simulink model "P2002_230207_MasterTest01"  (R2022b)
settings: Solver=VariableStepAuto  StartTime=0.0  StopTime=30  RelTol=1e-7
settings Model: PacingRate=0.100000  Creator=turib  LastModifiedBy=turib

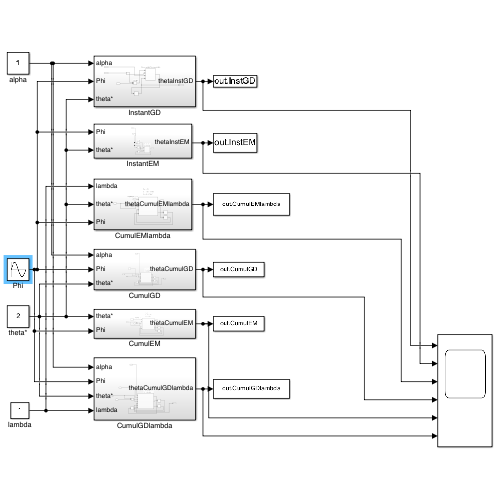
[thumbnail: Simulink's stored preview of the top-level diagram]
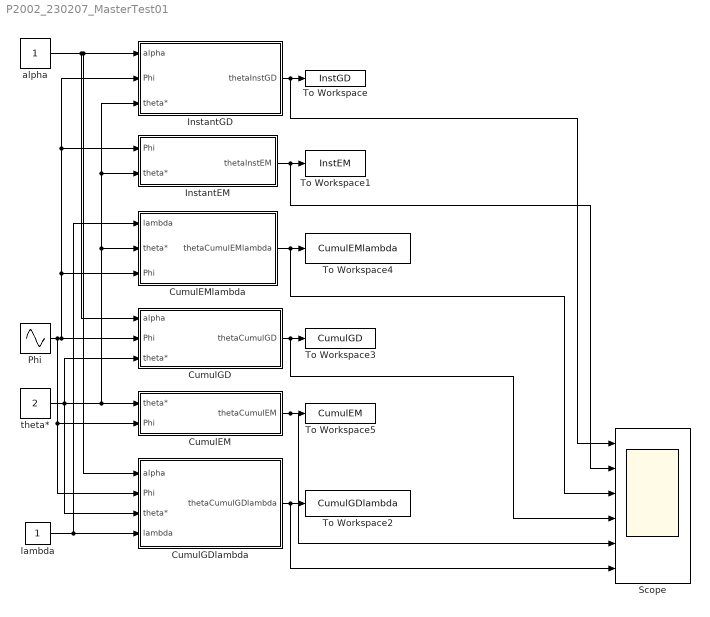
== system P2002_230207_MasterTest01 ==
  CumulEM : Subsystem
  CumulEMlambda : Subsystem
  CumulGD : Subsystem
  CumulGDlambda : Subsystem
  InstantEM : Subsystem
  InstantGD : Subsystem
  Phi : Sin  SampleTime=0
  Scope : Scope  NumInputPorts=6
  To Workspace : ToWorkspace  VariableName=InstGD  SampleTime=-1
  To Workspace1 : ToWorkspace  VariableName=InstEM  SampleTime=-1
  To Workspace2 : ToWorkspace  VariableName=CumulGDlambda  SampleTime=-1
  To Workspace3 : ToWorkspace  VariableName=CumulGD  SampleTime=-1
  To Workspace4 : ToWorkspace  VariableName=CumulEMlambda  SampleTime=-1
  To Workspace5 : ToWorkspace  VariableName=CumulEM  SampleTime=-1
  alpha : Constant
  lambda : Constant
  theta* : Constant  Value=2
  wires:
  lambda/1 -> CumulGDlambda/4(lambda), CumulEMlambda/1(lambda)
  alpha/1 -> InstantGD/1(alpha), CumulGDlambda/1(alpha), CumulGD/1(alpha)
  Phi/1 -> CumulEM/2(Phi), CumulGDlambda/2(Phi), CumulGD/2(Phi), InstantGD/2(Phi), InstantEM/1(Phi), CumulEMlambda/3(Phi)
  theta*/1 -> CumulGDlambda/3(theta*), InstantEM/2(theta*), InstantGD/3(theta*), CumulEMlambda/2(theta*), CumulEM/1(theta*), CumulGD/3(theta*)
  CumulEMlambda/1(thetaCumulEMlambda) -> Scope/3, To Workspace4/1
  InstantGD/1(thetaInstGD) -> Scope/1, To Workspace/1
  InstantEM/1(thetaInstEM) -> Scope/2, To Workspace1/1
  CumulGD/1(thetaCumulGD) -> Scope/4, To Workspace3/1
  CumulEM/1(thetaCumulEM) -> Scope/5, To Workspace5/1
  CumulGDlambda/1(thetaCumulGDlambda) -> Scope/6, To Workspace2/1

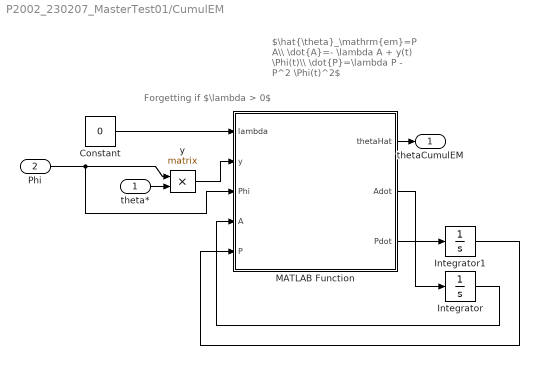
== system P2002_230207_MasterTest01/CumulEM ==
  note: $\hat{\theta}_\mathrm{em}=P A\\ \dot{A}=- \lambda A + y(t) \Phi(t)\\ \dot{P}=\lambda P - P^2 \Phi(t)^2$
  note: Forgetting if $\lambda > 0$
  theta* : Inport
  Phi : Inport  Port=2
  Constant : Constant  Value=0
  Integrator : Integrator  InitialCondition=1
  Integrator1 : Integrator  InitialCondition=1
  MATLAB Function : MATLAB Function  TreatAsAtomicUnit=on
  y : Product  Multiplication=Matrix(*)  OutDataTypeStr=double
  thetaCumulEM : Outport
  wires:
  theta*/1 -> y/2
  MATLAB Function/3(Pdot) -> Integrator1/1
  Integrator1/1 -> MATLAB Function/5(P)
  Integrator/1 -> MATLAB Function/4(A)
  Constant/1 -> MATLAB Function/1(lambda)
  y/1 -> MATLAB Function/2(y)
  MATLAB Function/2(Adot) -> Integrator/1
  MATLAB Function/1(thetaHat) -> thetaCumulEM/1
  Phi/1 -> y/1, MATLAB Function/3(Phi)

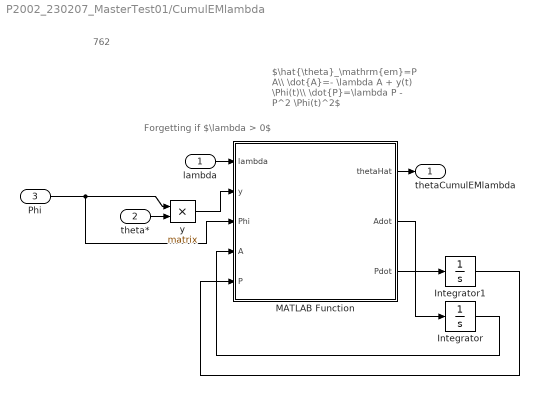
== system P2002_230207_MasterTest01/CumulEMlambda ==
  note: 762
  note: $\hat{\theta}_\mathrm{em}=P A\\ \dot{A}=- \lambda A + y(t) \Phi(t)\\ \dot{P}=\lambda P - P^2 \Phi(t)^2$
  note: Forgetting if $\lambda > 0$
  lambda : Inport
  theta* : Inport  Port=2
  Phi : Inport  Port=3
  Integrator : Integrator  InitialCondition=1
  Integrator1 : Integrator  InitialCondition=1
  MATLAB Function : MATLAB Function  TreatAsAtomicUnit=on
  y : Product  Multiplication=Matrix(*)  OutDataTypeStr=double
  thetaCumulEMlambda : Outport
  wires:
  theta*/1 -> y/2
  MATLAB Function/3(Pdot) -> Integrator1/1
  Integrator1/1 -> MATLAB Function/5(P)
  Integrator/1 -> MATLAB Function/4(A)
  lambda/1 -> MATLAB Function/1(lambda)
  y/1 -> MATLAB Function/2(y)
  MATLAB Function/2(Adot) -> Integrator/1
  MATLAB Function/1(thetaHat) -> thetaCumulEMlambda/1
  Phi/1 -> y/1, MATLAB Function/3(Phi)

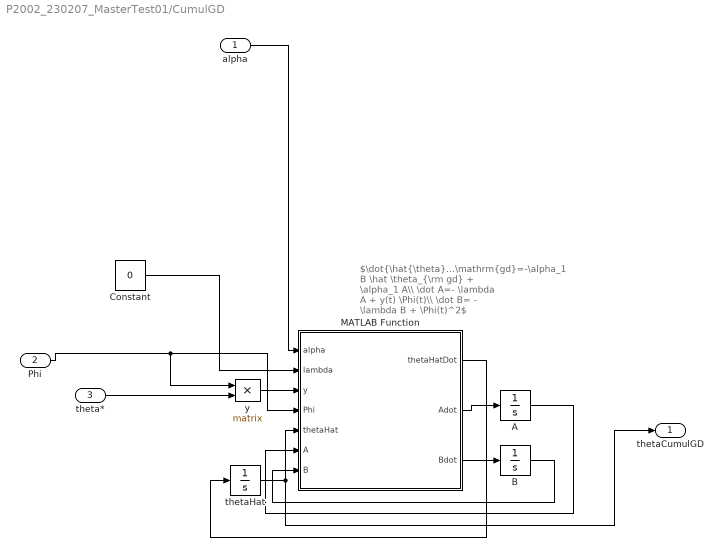
== system P2002_230207_MasterTest01/CumulGD ==
  note: $\dot{\hat{\theta}}_\mathrm{gd}=-\alpha_1 B \hat \theta_{\rm gd} + \alpha_1 A\\ \dot A=- \lambda A + y(t) \Phi(t)\\ \dot B= - \lambda B + \Phi(t)^2$
  alpha : Inport
  Phi : Inport  Port=2
  theta* : Inport  Port=3
  A : Integrator  InitialCondition=1
  B : Integrator  InitialCondition=1
  Constant : Constant  Value=0
  MATLAB Function : MATLAB Function  TreatAsAtomicUnit=on
  thetaHat : Integrator
  y : Product  Multiplication=Matrix(*)  OutDataTypeStr=double
  thetaCumulGD : Outport
  wires:
  thetaHat/1 -> thetaCumulGD/1, MATLAB Function/5(thetaHat)
  B/1 -> MATLAB Function/7(B)
  MATLAB Function/3(Bdot) -> B/1
  A/1 -> MATLAB Function/6(A)
  theta*/1 -> y/2
  MATLAB Function/1(thetaHatDot) -> thetaHat/1
  y/1 -> MATLAB Function/3(y)
  MATLAB Function/2(Adot) -> A/1
  Phi/1 -> MATLAB Function/4(Phi), y/1
  alpha/1 -> MATLAB Function/1(alpha)
  Constant/1 -> MATLAB Function/2(lambda)

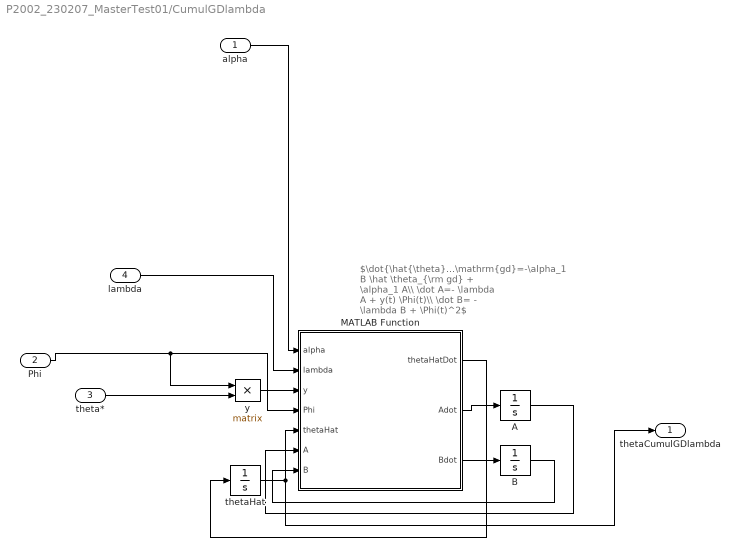
== system P2002_230207_MasterTest01/CumulGDlambda ==
  note: $\dot{\hat{\theta}}_\mathrm{gd}=-\alpha_1 B \hat \theta_{\rm gd} + \alpha_1 A\\ \dot A=- \lambda A + y(t) \Phi(t)\\ \dot B= - \lambda B + \Phi(t)^2$
  alpha : Inport
  Phi : Inport  Port=2
  theta* : Inport  Port=3
  lambda : Inport  Port=4
  A : Integrator  InitialCondition=1
  B : Integrator  InitialCondition=1
  MATLAB Function : MATLAB Function  TreatAsAtomicUnit=on
  thetaHat : Integrator
  y : Product  Multiplication=Matrix(*)  OutDataTypeStr=double
  thetaCumulGDlambda : Outport
  wires:
  thetaHat/1 -> thetaCumulGDlambda/1, MATLAB Function/5(thetaHat)
  B/1 -> MATLAB Function/7(B)
  MATLAB Function/3(Bdot) -> B/1
  A/1 -> MATLAB Function/6(A)
  theta*/1 -> y/2
  MATLAB Function/1(thetaHatDot) -> thetaHat/1
  y/1 -> MATLAB Function/3(y)
  MATLAB Function/2(Adot) -> A/1
  Phi/1 -> MATLAB Function/4(Phi), y/1
  lambda/1 -> MATLAB Function/2(lambda)
  alpha/1 -> MATLAB Function/1(alpha)

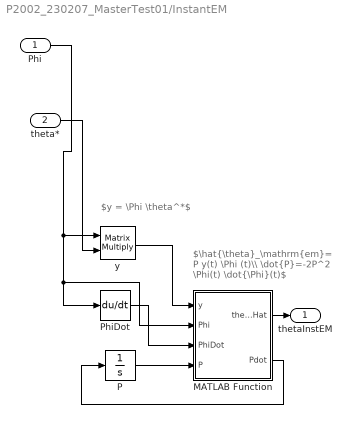
== system P2002_230207_MasterTest01/InstantEM ==
  note: $y = \Phi \theta^*$
  note: $\hat{\theta}_\mathrm{em}= P y(t) \Phi (t)\\ \dot{P}=-2P^2 \Phi(t) \dot{\Phi}(t)$
  Phi : Inport
  theta* : Inport  Port=2
  MATLAB Function : MATLAB Function  TreatAsAtomicUnit=on
  P : Integrator  InitialCondition=1
  PhiDot : Derivative
  y : Product  Multiplication=Matrix(*)  OutDataTypeStr=double
  thetaInstEM : Outport
  wires:
  Phi/1 -> y/1, MATLAB Function/2(Phi), PhiDot/1
  P/1 -> MATLAB Function/4(P)
  PhiDot/1 -> MATLAB Function/3(PhiDot)
  theta*/1 -> y/2
  MATLAB Function/2(Pdot) -> P/1
  y/1 -> MATLAB Function/1(y)
  MATLAB Function/1(thetaHat) -> thetaInstEM/1

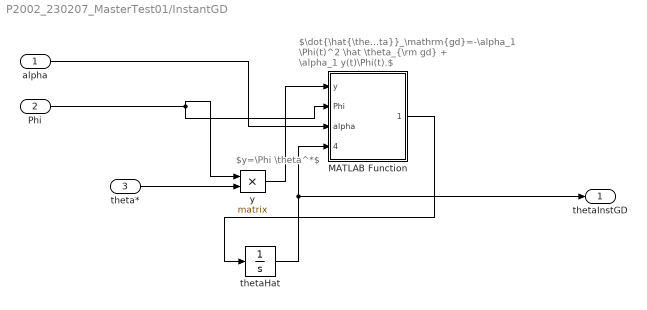
== system P2002_230207_MasterTest01/InstantGD ==
  note: $y=\Phi \theta^*$
  note: $\dot{\hat{\theta}}_\mathrm{gd}=-\alpha_1 \Phi(t)^2 \hat \theta_{\rm gd} + \alpha_1 y(t)\Phi(t).$
  alpha : Inport
  Phi : Inport  Port=2
  theta* : Inport  Port=3
  MATLAB Function : MATLAB Function  TreatAsAtomicUnit=on
  thetaHat : Integrator
  y : Product  Multiplication=Matrix(*)  OutDataTypeStr=double
  thetaInstGD : Outport
  wires:
  theta*/1 -> y/2
  MATLAB Function/1(thetaHatDot) -> thetaHat/1
  thetaHat/1 -> thetaInstGD/1, MATLAB Function/4(thetaHat)
  alpha/1 -> MATLAB Function/3(alpha)
  Phi/1 -> y/1, MATLAB Function/2(Phi)
  y/1 -> MATLAB Function/1(y)

== matlab function P2002_230207_MasterTest01/InstantEM/MATLAB Function ==
  data: thetaHat output; y input; Phi input; PhiDot input; Pdot output; P input
function [thetaHat, Pdot] = fcn(y, Phi, PhiDot, P)
thetaHat = P * y * Phi;
Pdot = - 2 * (P ^ 2) * Phi * PhiDot;
end

== matlab function P2002_230207_MasterTest01/InstantGD/MATLAB Function ==
  data: thetaHatDot output; y input; Phi input; alpha input; thetaHat input
function thetaHatDot  = fcn(y, Phi, alpha, thetaHat)
thetaHatDot = - alpha * (Phi ^ 2) * thetaHat + alpha * y * Phi;
end

== matlab function P2002_230207_MasterTest01/CumulGDlambda/MATLAB Function ==
  data: alpha input; thetaHatDot output; lambda input; Adot output; y input; Phi input; thetaHat input; A input; B input; Bdot output
function [thetaHatDot, Adot, Bdot] = fcn(alpha, lambda, y, Phi, ...
    thetaHat, A, B)

thetaHatDot = - alpha * B * thetaHat + alpha * A;
Adot = - lambda * A + y * Phi;
Bdot = - lambda * B + Phi ^ 2;

end

== matlab function P2002_230207_MasterTest01/CumulGD/MATLAB Function ==
  data: alpha input; thetaHatDot output; lambda input; Adot output; y input; Phi input; thetaHat input; A input; B input; Bdot output
function [thetaHatDot, Adot, Bdot] = fcn(alpha, lambda, y, Phi, ...
    thetaHat, A, B)

thetaHatDot = - alpha * B * thetaHat + alpha * A;
Adot = - lambda * A + y * Phi;
Bdot = - lambda * B + Phi ^ 2;

end

== matlab function P2002_230207_MasterTest01/CumulEMlambda/MATLAB Function ==
  data: thetaHat output; lambda input; Adot output; y input; Phi input; A input; P input; Pdot output
function [thetaHat, Adot, Pdot] = fcn(lambda, y, Phi, ...
    A, P)

thetaHat = P * A;
Adot = - lambda * A + y * Phi;
Pdot = lambda * P - P ^ 2 * Phi ^ 2;
% B = inv(P);
% Jder = -2 * (A - B * thetaHat);

end

== matlab function P2002_230207_MasterTest01/CumulEM/MATLAB Function ==
  data: thetaHat output; lambda input; Adot output; y input; Phi input; A input; P input; Pdot output
function [thetaHat, Adot, Pdot] = fcn(lambda, y, Phi, ...
    A, P)

thetaHat = P * A;
Adot = - lambda * A + y * Phi;
Pdot = lambda * P - P ^ 2 * Phi ^ 2;
% B = inv(P);
% Jder = -2 * (A - B * thetaHat);

end
